simulink model "sampleModel2004"  (R2023a)
settings: Solver=VariableStepAuto  StartTime=0.0  StopTime=10.0  RelTol=1e-3
libraries: simulink x5, hdlsllib x3
settings Model: Creator=user1  LastModifiedBy=user1

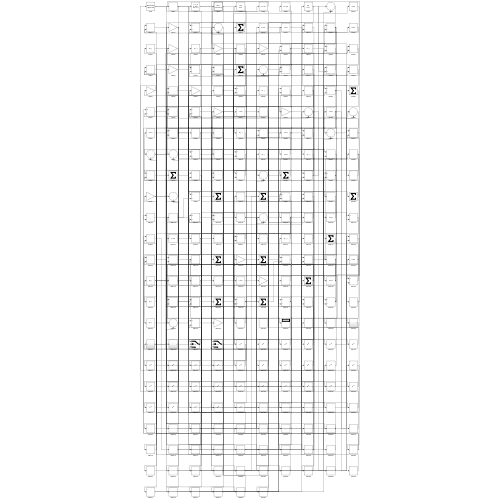
[thumbnail: Simulink's stored preview of the top-level diagram]
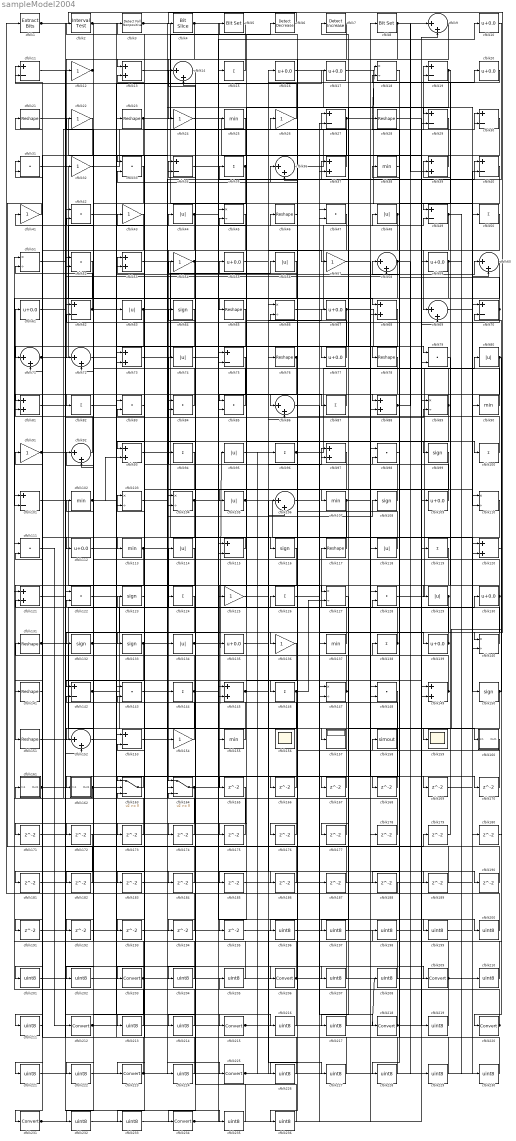
== system sampleModel2004 ==
  cfblk1 : simulink/Logic and Bit Operations/Extract Bits  bitsToExtract=Upper half  numBits=8  bitIdxRange=[0 7]  outScalingMode=Preserve fixed-point scaling
      settings: LibrarySourceBlock=|
      | hdlsllib/Logic and Bit
      | Operations/Extract Bits
  cfblk{10,16..17,20,55,59,61,67,77,109,112,130,135,139} (14 alike) : Bias  Bias=0.0  SaturateOnIntegerOverflow=off
  cfblk{15,35,50,82,87,94,96,100,119,124,126,138,144,146} (14 alike) : Sum  Inputs=+
  cfblk{11,19,27,29..30,34,40,49,62,70,75,101,115,142,153} (15 alike) : Sum  Inputs=+-
  cfblk{25,38,90,102,107,113,137,155} (8 alike) : MinMax
  cfblk{18,45,51,66,89,103..104,110,127,140,147} (11 alike) : Product  Inputs=*/  RndMeth=Zero  SaturateOnIntegerOverflow=on
  cfblk{44,48,56,63,74,80,95,105,114,118,129,134} (12 alike) : Abs  SaturateOnIntegerOverflow=off
  cfblk{9,14,36,58,60,69,71..72,86,92,106,152} (12 alike) : Sum  Inputs=|++
  cfblk{64,99,108,116,123,132..133,150} (8 alike) : Signum
  cfblk{31,33,42,47,52,79,83..85,98,111,122,128,143,148} (15 alike) : DotProduct  OutDataTypeStr=Inherit: Inherit via internal rule
  cfblk{21,23,28,46,65,76,78,117,131,141,151} (11 alike) : Reshape
  cfblk{12,22,24,26,32,41,43,54,57,91,125,136,154} (13 alike) : Gain
  cfblk{13,37,39,53,68,73,81,88,93,97,120..121,145,149} (14 alike) : Sum
  cfblk156 : Scope
      settings: Floating=on
  cfblk157 : Display
  cfblk158 : ToWorkspace  VariableName=simout  SaveFormat=Timeseries  SampleTime=-1
  cfblk159 : Scope
  cfblk160 : Subsystem
      settings: LibrarySourceBlock=|
      | hdlsllib/Ports &
      | Subsystems/Subsystem
  cfblk161 : Subsystem
      settings: LibrarySourceBlock=|
      | hdlsllib/Ports &
      | Subsystems/Subsystem
  cfblk162 : Subsystem
      settings: LibrarySourceBlock=|
      | hdlsllib/Ports &
      | Subsystems/Subsystem
  cfblk163 : Switch  SaturateOnIntegerOverflow=off  InputSameDT=off
  cfblk164 : Switch  SaturateOnIntegerOverflow=off  InputSameDT=off
  cfblk{165..195} (31 alike) : Delay  SampleTime=1
  cfblk{196..202,204..205,207..208,210..211,213..214,216..217,219,221..222,224,226..230,232..233,235..236} (30 alike) : DataTypeConversion  OutDataTypeStr=uint8  SaturateOnIntegerOverflow=off  RndMeth=Floor
  cfblk2 : hdlsllib/Logic and Bit Operations/Interval Test  IntervalClosedRight=on  uplimit=0.5  IntervalClosedLeft=on  lowlimit=-0.5  OutDataTypeStr=boolean
  cfblk{203,206,209,212,215,218,220,223,225,231,234} (11 alike) : DataTypeConversion  SaturateOnIntegerOverflow=off  RndMeth=Floor
  cfblk3 : hdlsllib/Logic and Bit Operations/Detect Fall Nonpositive  vinit=0  OutDataTypeStr=boolean
  cfblk4 : hdlsllib/Logic and Bit Operations/Bit Slice  lidx=7  ridx=0
  cfblk5 : simulink/Logic and Bit Operations/Bit Set  iBit=0
      settings: LibrarySourceBlock=|
      | hdlsllib/Logic and Bit
      | Operations/Bit Set
  cfblk6 : simulink/Logic and Bit Operations/Detect Decrease  vinit=0.0  OutDataTypeStr=boolean
      settings: LibrarySourceBlock=|
      | hdlsllib/Logic and Bit
      | Operations/Detect
      | Decrease
  cfblk7 : simulink/Logic and Bit Operations/Detect Increase  vinit=0.0  OutDataTypeStr=boolean
      settings: LibrarySourceBlock=|
      | hdlsllib/Logic and Bit
      | Operations/Detect
      | Increase
  cfblk8 : simulink/Logic and Bit Operations/Bit Set  iBit=0
      settings: LibrarySourceBlock=|
      | hdlsllib/Logic and Bit
      | Operations/Bit Set
  wires:
  cfblk163/1 -> cfblk162/1(In1)
  cfblk162/1(Out1) -> cfblk27/1, cfblk49/2
  cfblk71/1 -> cfblk44/1, cfblk149/2
  cfblk142/1 -> cfblk130/1, cfblk157/1
  cfblk53/1 -> cfblk116/1
  cfblk31/1 -> cfblk65/1
  cfblk10/1 -> cfblk35/1
  cfblk164/1 -> cfblk95/1, cfblk201/1
  cfblk107/1 -> cfblk132/1, cfblk30/2, cfblk183/1, cfblk185/1
  cfblk147/1 -> cfblk102/1, cfblk197/1
  cfblk83/1 -> cfblk203/1
  cfblk19/1 -> cfblk77/1, cfblk49/1, cfblk195/1
  cfblk85/1 -> cfblk41/1
  cfblk128/1 -> cfblk80/1
  cfblk44/1 -> cfblk164/1, cfblk79/2
  cfblk47/1 -> cfblk231/1
  cfblk152/1 -> cfblk23/1
  cfblk50/1 -> cfblk69/1
  cfblk89/1 -> cfblk22/1, cfblk175/1
  cfblk96/1 -> cfblk50/1, cfblk166/1
  cfblk73/1 -> cfblk56/1
  cfblk126/1 -> cfblk218/1
  cfblk1/1 -> cfblk140/1, cfblk135/1
  cfblk66/1 -> cfblk48/1
  cfblk37/1 -> cfblk3/1
  cfblk63/1 -> cfblk110/2, cfblk171/1
  cfblk137/1 -> cfblk114/1
  cfblk132/1 -> cfblk17/1, cfblk184/1
  cfblk116/1 -> cfblk155/1
  cfblk22/1 -> cfblk72/1
  cfblk16/1 -> cfblk90/1
  cfblk149/1 -> cfblk39/1, cfblk64/1
  cfblk17/1 -> cfblk110/1
  cfblk146/1 -> cfblk154/1, cfblk127/2
  cfblk2/1 -> cfblk125/1, cfblk100/1, cfblk202/1
  cfblk109/1 -> cfblk74/1
  cfblk59/1 -> cfblk72/2, cfblk145/2, cfblk210/1
  cfblk33/1 -> cfblk82/1
  cfblk32/1 -> cfblk26/1
  cfblk92/1 -> cfblk61/1
  cfblk23/1 -> cfblk6/1, cfblk191/1
  cfblk154/1 -> cfblk92/1
  cfblk138/1 -> cfblk117/1, cfblk34/1
  cfblk24/1 -> cfblk109/1
  cfblk82/1 -> cfblk63/1
  cfblk80/1 -> cfblk159/1, cfblk133/1
  cfblk26/1 -> cfblk11/1
  cfblk153/1 -> cfblk225/1
  cfblk120/1 -> cfblk220/1
  cfblk111/1 -> cfblk212/1
  cfblk145/1 -> cfblk16/1, cfblk67/1
  cfblk121/1 -> cfblk215/1
  cfblk60/1 -> cfblk136/1
  cfblk134/1 -> cfblk115/1, cfblk34/2
  cfblk15/1 -> cfblk13/1
  cfblk118/1 -> cfblk2/1
  cfblk140/1 -> cfblk5/1
  cfblk151/1 -> cfblk27/2
  cfblk99/1 -> cfblk107/1
  cfblk55/1 -> cfblk57/1
  cfblk27/1 -> cfblk18/1, cfblk85/1
  cfblk43/1 -> cfblk81/1
  cfblk95/1 -> cfblk20/1
  cfblk52/1 -> cfblk71/1
  cfblk133/1 -> cfblk104/1, cfblk142/1
  cfblk129/1 -> cfblk134/1, cfblk148/2
  cfblk160/1(Out1) -> cfblk158/1
  cfblk90/1 -> cfblk55/1
  cfblk62/1 -> cfblk78/1, cfblk31/1, cfblk99/1
  cfblk135/1 -> cfblk40/1
  cfblk3/1 -> cfblk119/1, cfblk29/1
  cfblk115/1 -> cfblk113/1
  cfblk4/1 -> cfblk32/1, cfblk79/1
  cfblk35/1 -> cfblk115/2, cfblk163/2
  cfblk76/1 -> cfblk146/1, cfblk86/1
  cfblk5/1 -> cfblk24/1
  cfblk155/1 -> cfblk103/1
  cfblk21/1 -> cfblk144/1
  cfblk8/1 -> cfblk75/2, cfblk39/2
  cfblk36/1 -> cfblk19/1
  cfblk103/1 -> cfblk37/1
  cfblk112/1 -> cfblk60/1
  cfblk123/1 -> cfblk223/1
  cfblk69/1 -> cfblk60/2
  cfblk12/1 -> cfblk152/1, cfblk192/1
  cfblk29/1 -> cfblk73/2
  cfblk54/1 -> cfblk30/1, cfblk10/1, cfblk233/1
  cfblk45/1 -> cfblk52/2
  cfblk113/1 -> cfblk43/1, cfblk108/1, cfblk211/1
  cfblk100/1 -> cfblk54/1
  cfblk72/1 -> cfblk46/1
  cfblk79/1 -> cfblk129/1
  cfblk58/1 -> cfblk112/1, cfblk229/1
  cfblk150/1 -> cfblk70/2, cfblk217/1
  cfblk104/1 -> cfblk141/1, cfblk169/1
  cfblk67/1 -> cfblk149/1, cfblk236/1
  cfblk143/1 -> cfblk206/1
  cfblk139/1 -> cfblk11/2, cfblk21/1
  cfblk130/1 -> cfblk122/2, cfblk92/2, cfblk127/1, cfblk194/1
  cfblk61/1 -> cfblk68/1
  cfblk84/1 -> cfblk53/1
  cfblk48/1 -> cfblk94/1, cfblk85/2
  cfblk125/1 -> cfblk97/1
  cfblk56/1 -> cfblk101/2
  cfblk25/1 -> cfblk93/1
  cfblk20/1 -> cfblk18/2
  cfblk93/1 -> cfblk105/1
  cfblk6/1 -> cfblk4/1
  cfblk91/1 -> cfblk12/1, cfblk58/2
  cfblk70/1 -> cfblk28/1, cfblk62/2
  cfblk105/1 -> cfblk150/1, cfblk190/1
  cfblk9/1 -> cfblk36/2
  cfblk14/1 -> cfblk234/1
  cfblk38/1 -> cfblk88/1
  cfblk74/1 -> cfblk87/1
  cfblk114/1 -> cfblk151/1
  cfblk81/1 -> cfblk145/1
  cfblk88/1 -> cfblk58/1, cfblk9/1
  cfblk77/1 -> cfblk45/2
  cfblk131/1 -> cfblk160/1(In1), cfblk69/2, cfblk235/1
  cfblk39/1 -> cfblk33/1
  cfblk144/1 -> cfblk25/1, cfblk91/1, cfblk193/1
  cfblk49/1 -> cfblk104/2, cfblk230/1
  cfblk161/1(Out1) -> cfblk89/2, cfblk189/1
  cfblk101/1 -> cfblk147/2
  cfblk102/1 -> cfblk93/2, cfblk216/1
  cfblk108/1 -> cfblk13/2
  cfblk117/1 -> cfblk33/2
  cfblk97/1 -> cfblk124/1
  cfblk86/1 -> cfblk139/1
  cfblk141/1 -> cfblk81/2
  cfblk87/1 -> cfblk66/2
  cfblk75/1 -> cfblk84/2
  cfblk51/1 -> cfblk209/1
  cfblk148/1 -> cfblk163/1
  cfblk136/1 -> cfblk165/1
  cfblk166/1 -> cfblk103/2
  cfblk42/1 -> cfblk167/1
  cfblk167/1 -> cfblk147/1
  cfblk18/1 -> cfblk168/1
  cfblk168/1 -> cfblk52/1
  cfblk169/1 -> cfblk140/2
  cfblk57/1 -> cfblk170/1
  cfblk170/1 -> cfblk36/1
  cfblk171/1 -> cfblk75/1
  cfblk110/1 -> cfblk172/1
  cfblk64/1 -> cfblk173/1
  cfblk173/1 -> cfblk71/2
  cfblk68/1 -> cfblk174/1
  cfblk174/1 -> cfblk164/2
  cfblk175/1 -> cfblk73/1
  cfblk46/1 -> cfblk176/1
  cfblk176/1 -> cfblk84/1
  cfblk127/1 -> cfblk177/1
  cfblk177/1 -> cfblk45/1
  cfblk178/1 -> cfblk101/1
  cfblk41/1 -> cfblk179/1
  cfblk179/1 -> cfblk19/2
  cfblk78/1 -> cfblk181/1
  cfblk181/1 -> cfblk88/2
  cfblk65/1 -> cfblk182/1
  cfblk182/1 -> cfblk62/1
  cfblk183/1 -> cfblk70/1
  cfblk184/1 -> cfblk122/1
  cfblk185/1 -> cfblk37/2
  cfblk13/1 -> cfblk186/1
  cfblk186/1 -> cfblk66/1
  cfblk187/1 -> cfblk164/3
  cfblk40/1 -> cfblk188/1
  cfblk188/1 -> cfblk1/1
  cfblk189/1 -> cfblk97/2
  cfblk190/1 -> cfblk53/2
  cfblk191/1 -> cfblk152/2
  cfblk192/1 -> cfblk86/2
  cfblk193/1 -> cfblk9/2
  cfblk194/1 -> cfblk142/2
  cfblk7/1 -> cfblk196/1
  cfblk196/1 -> cfblk118/1
  cfblk197/1 -> cfblk7/1
  cfblk180/1 -> cfblk198/1
  cfblk198/1 -> cfblk128/2
  cfblk34/1 -> cfblk199/1
  cfblk199/1 -> cfblk180/1
  cfblk106/1 -> cfblk200/1
  cfblk200/1 -> cfblk128/1
  cfblk201/1 -> cfblk106/1
  cfblk202/1 -> cfblk106/2
  cfblk203/1 -> cfblk40/2, cfblk42/2, cfblk232/1
  cfblk30/1 -> cfblk204/1
  cfblk204/1 -> cfblk83/1
  cfblk205/1 -> cfblk83/2
  cfblk206/1 -> cfblk178/1, cfblk131/1
  cfblk11/1 -> cfblk207/1
  cfblk207/1 -> cfblk143/1
  cfblk208/1 -> cfblk143/2
  cfblk209/1 -> cfblk205/1, cfblk161/1(In1)
  cfblk210/1 -> cfblk51/1
  cfblk211/1 -> cfblk51/2
  cfblk212/1 -> cfblk208/1, cfblk8/1
  cfblk94/1 -> cfblk213/1
  cfblk213/1 -> cfblk111/1
  cfblk165/1 -> cfblk214/1
  cfblk214/1 -> cfblk111/2
  cfblk215/1 -> cfblk59/1, cfblk137/1
  cfblk216/1 -> cfblk121/1
  cfblk217/1 -> cfblk121/2
  cfblk218/1 -> cfblk138/1, cfblk148/1
  cfblk28/1 -> cfblk219/1
  cfblk219/1 -> cfblk126/1
  cfblk220/1 -> cfblk163/3, cfblk38/1
  cfblk172/1 -> cfblk221/1
  cfblk221/1 -> cfblk120/1
  cfblk124/1 -> cfblk222/1
  cfblk222/1 -> cfblk120/2
  cfblk223/1 -> cfblk31/2, cfblk76/1
  cfblk122/1 -> cfblk224/1
  cfblk224/1 -> cfblk123/1
  cfblk225/1 -> cfblk29/2, cfblk96/1
  cfblk119/1 -> cfblk226/1
  cfblk226/1 -> cfblk153/1
  cfblk195/1 -> cfblk227/1
  cfblk227/1 -> cfblk153/2
  cfblk98/1 -> cfblk228/1
  cfblk228/1 -> cfblk42/1
  cfblk229/1 -> cfblk98/1
  cfblk230/1 -> cfblk98/2
  cfblk231/1 -> cfblk187/1, cfblk15/1
  cfblk232/1 -> cfblk47/1
  cfblk233/1 -> cfblk47/2
  cfblk234/1 -> cfblk89/1, cfblk68/2
  cfblk235/1 -> cfblk14/1
  cfblk236/1 -> cfblk14/2

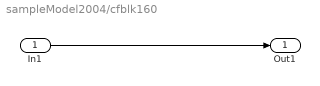
== system sampleModel2004/cfblk160 ==
  In1 : Inport
  Out1 : Outport
  wires:
  In1/1 -> Out1/1

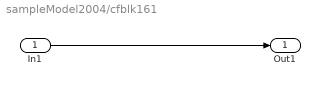
== system sampleModel2004/cfblk161 ==
  In1 : Inport
  Out1 : Outport
  wires:
  In1/1 -> Out1/1

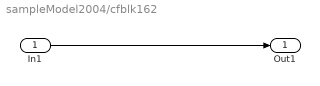
== system sampleModel2004/cfblk162 ==
  In1 : Inport
  Out1 : Outport
  wires:
  In1/1 -> Out1/1
